simulink model "OpenLoop_NonLin"  (Simulink 10.1)
settings: Solver=ode45  StartTime=0.0  StopTime=100  RelTol=1e-3  EnableMultiTasking=on
settings Model: Creator=mchi9aa4  LastModifiedBy=shita
settings DataIOCC: LimitDataPoints=on  SignalLoggingSaveFormat=ModelDataLogs  Refine=10
settings OptimizationCC: ExpressionDepthLimit=2147483647
settings DebuggingCC: SolverPrmCheckMsg=warning  FcnCallInpInsideContextMsg=warning  StateNameClashWarn=warning
settings GRTTargetCC: CombineOutputUpdateFcns=on  GRTInterface=off

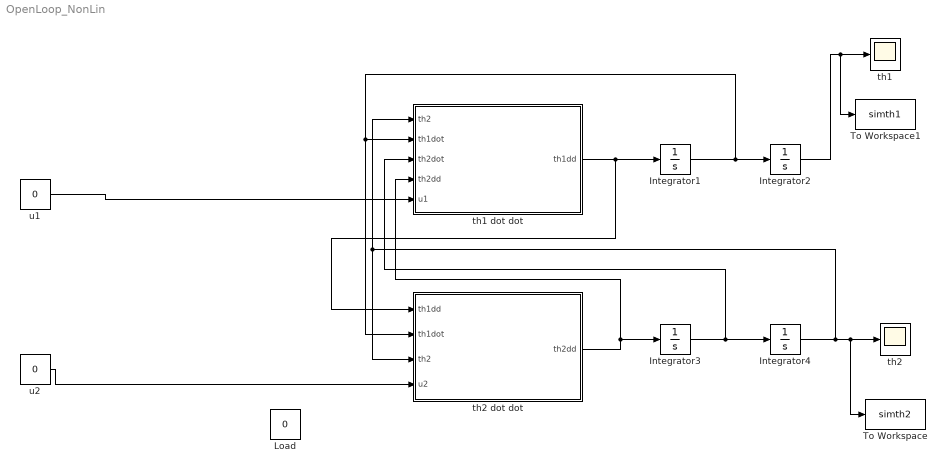
== system OpenLoop_NonLin ==
  Integrator1 : Integrator
  Integrator2 : Integrator  InitialCondition=pi/2.1
  Integrator3 : Integrator
  Integrator4 : Integrator
  Load : Constant  Value=0
  To Workspace : ToWorkspace  VariableName=simth2  SampleTime=-1
  To Workspace1 : ToWorkspace  VariableName=simth1  SampleTime=-1
  th1 : Scope
  th1 dot dot : MATLAB Function  TreatAsAtomicUnit=on
  th2 : Scope
  th2 dot dot : MATLAB Function  TreatAsAtomicUnit=on
  u1 : Constant  Value=0
  u2 : Constant  Value=0
  wires:
  th1 dot dot/1(th1dd) -> th2 dot dot/1(th1dd), Integrator1/1
  Integrator1/1 -> Integrator2/1, th2 dot dot/2(th1dot), th1 dot dot/2(th1dot)
  th2 dot dot/1(th2dd) -> th1 dot dot/4(th2dd), Integrator3/1
  Integrator3/1 -> Integrator4/1, th1 dot dot/3(th2dot)
  Integrator2/1 -> th1/1, To Workspace1/1
  Integrator4/1 -> th2 dot dot/3(th2), th1 dot dot/1(th2), th2/1, To Workspace/1
  u2/1 -> th2 dot dot/4(u2)
  u1/1 -> th1 dot dot/5(u1)

== matlab function th2 dot dot ==
  data: th1dd input double; th1dot input double; th2 input double; th2dd output double; u2 input double
function th2dd = fcn(th1dd, th1dot, th2, u2)
%#codegen
m1 = 20;
m2 = 10;
L1 = 1;
L2 = 1;
I1 = 0.8;
I2 = 0.2;
th2dotdot = (u2 - I2*th1dd - L2^2*m2*th1dd - L1*L2*m2*th1dot^2*sin(th2) - L1*L2*m2*th1dd*cos(th2))/(L2^2*m2 + I2) ;
th2dd = th2dotdot;

== matlab function th1 dot dot ==
  data: th2 input double; th1dot input double; th2dot input double; th2dd input double; th1dd output double; u1 input double
function th1dd = fcn(th2,th1dot,  th2dot, th2dd, u1)
%#codegen
m1 = 20;
m2 = 10;
L1 = 1;
L2 = 1;
I1 = 0.8;
I2 = 0.2;
th1dotdot = (u1 + L1*L2*m2*th2dot*sin(th2)*(2*th1dot + th2dot) - th2dd(m2*L2^2 + L1*m2*cos(th2)*L2 + I2)) / (I1 + I2 + L1^2*m1 + L1^2*m2 + L2^2*m2 + 2*L1*L2*m2*cos(th2));
th1dd = th1dotdot;
